simulink model "Parallel_n49"  (R2012b)
settings: Solver=VariableStepDiscrete  StartTime=0.0  StopTime=TotalIterations  RelTol=1e-3
values from neighbouring files (symbols this model uses):
  bp = 12    [ConfigValidate.m]
  bpSNMemory = bp    (= 12)    [ConfigValidate.m]
  IterationsOrdering = 4000    [ConfigValidate.m]
  MaxCoordDistance = (abs(max(wx) - min(wx))+abs(max(wy) - min(wy)))^2    [ConfigValidate.m]
  N_limit = 0.01    [ConfigValidate.m]
  nBits = 9    [ConfigValidate.m]
  nBitsNSmemories = (ceil(log2(TotalIterations)))    [ConfigValidate.m]
  S_limit = 1    [ConfigValidate.m]
  SourceNodes = 2000    [ConfigValidate.m]
  ts = 1    [ConfigValidate.m]
  w1 = rand(1,Neurons)    [ConfigValidate.m]
  w2 = rand(1,Neurons)    [ConfigValidate.m]
  wx = zeros(1,Neurons)    [ConfigValidate.m]
  wy = zeros(1,Neurons)    [ConfigValidate.m]
  x1 = rand(SourceNodes,1)    [ConfigValidate.m]
  x2 = rand(SourceNodes,1)    [ConfigValidate.m]
libraries: xbsIndex_r4 x4147, dspsrcs4 x2, dspstat3 x2
(part 2 of 19)

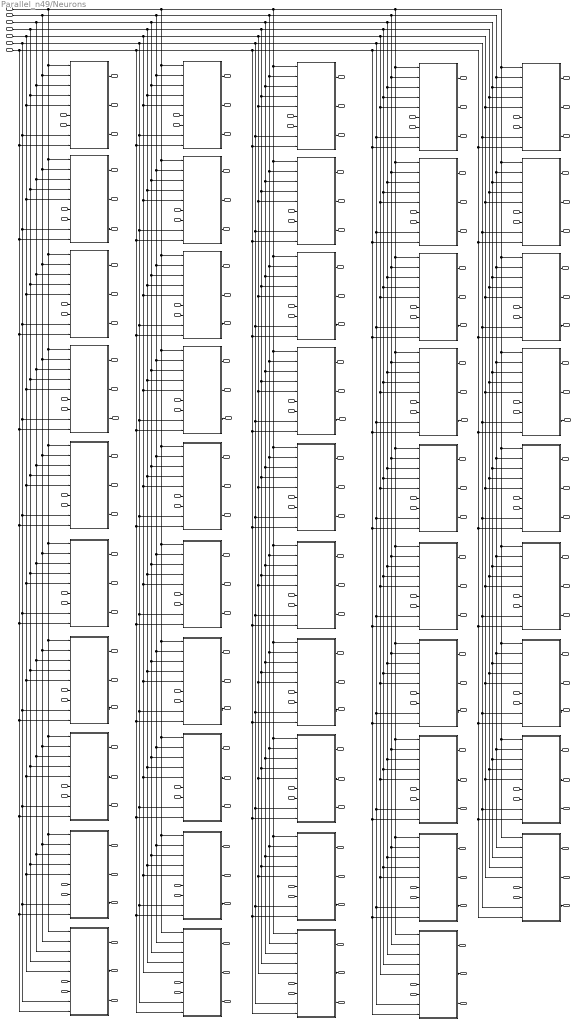
== system Parallel_n49/Neurons ==
  vX11 : Inport
  vX12 : Inport  Port=2
  S : Inport  Port=3
  N : Inport  Port=4
  memControl : Inport  Port=5
  wx_win : Inport  Port=6
  wy_win : Inport  Port=7
  wx1 : Inport  Port=8
  wy1 : Inport  Port=9
  wx2 : Inport  Port=10
  wy2 : Inport  Port=11
  wx3 : Inport  Port=12
  wy3 : Inport  Port=13
  wx4 : Inport  Port=14
  wy4 : Inport  Port=15
  wx5 : Inport  Port=16
  wy5 : Inport  Port=17
  wx6 : Inport  Port=18
  wy6 : Inport  Port=19
  wx7 : Inport  Port=20
  wy7 : Inport  Port=21
  wx8 : Inport  Port=22
  wy8 : Inport  Port=23
  wx9 : Inport  Port=24
  wy9 : Inport  Port=25
  wx10 : Inport  Port=26
  wy10 : Inport  Port=27
  wx11 : Inport  Port=28
  wy11 : Inport  Port=29
  wx12 : Inport  Port=30
  wy12 : Inport  Port=31
  wx13 : Inport  Port=32
  wy13 : Inport  Port=33
  wx14 : Inport  Port=34
  wy14 : Inport  Port=35
  wx15 : Inport  Port=36
  wy15 : Inport  Port=37
  wx16 : Inport  Port=38
  wy16 : Inport  Port=39
  wx17 : Inport  Port=40
  wy17 : Inport  Port=41
  wx18 : Inport  Port=42
  wy18 : Inport  Port=43
  wx19 : Inport  Port=44
  wy19 : Inport  Port=45
  wx20 : Inport  Port=46
  wy20 : Inport  Port=47
  wx21 : Inport  Port=48
  wy21 : Inport  Port=49
  wx22 : Inport  Port=50
  wy22 : Inport  Port=51
  wx23 : Inport  Port=52
  wy23 : Inport  Port=53
  wx24 : Inport  Port=54
  wy24 : Inport  Port=55
  wx25 : Inport  Port=56
  wy25 : Inport  Port=57
  wx26 : Inport  Port=58
  wy26 : Inport  Port=59
  wx27 : Inport  Port=60
  wy27 : Inport  Port=61
  wx28 : Inport  Port=62
  wy28 : Inport  Port=63
  wx29 : Inport  Port=64
  wy29 : Inport  Port=65
  wx30 : Inport  Port=66
  wy30 : Inport  Port=67
  wx31 : Inport  Port=68
  wy31 : Inport  Port=69
  wx32 : Inport  Port=70
  wy32 : Inport  Port=71
  wx33 : Inport  Port=72
  wy33 : Inport  Port=73
  wx34 : Inport  Port=74
  wy34 : Inport  Port=75
  wx35 : Inport  Port=76
  wy35 : Inport  Port=77
  wx36 : Inport  Port=78
  wy36 : Inport  Port=79
  wx37 : Inport  Port=80
  wy37 : Inport  Port=81
  wx38 : Inport  Port=82
  wy38 : Inport  Port=83
  wx39 : Inport  Port=84
  wy39 : Inport  Port=85
  wx40 : Inport  Port=86
  wy40 : Inport  Port=87
  wx41 : Inport  Port=88
  wy41 : Inport  Port=89
  wx42 : Inport  Port=90
  wy42 : Inport  Port=91
  wx43 : Inport  Port=92
  wy43 : Inport  Port=93
  wx44 : Inport  Port=94
  wy44 : Inport  Port=95
  wx45 : Inport  Port=96
  wy45 : Inport  Port=97
  wx46 : Inport  Port=98
  wy46 : Inport  Port=99
  wx47 : Inport  Port=100
  wy47 : Inport  Port=101
  wx48 : Inport  Port=102
  wy48 : Inport  Port=103
  wx49 : Inport  Port=104
  wy49 : Inport  Port=105
  Neuron1 : Subsystem
  Neuron10 : Subsystem
  Neuron11 : Subsystem
  Neuron12 : Subsystem
  Neuron13 : Subsystem
  Neuron14 : Subsystem
  Neuron15 : Subsystem
  Neuron16 : Subsystem
  Neuron17 : Subsystem
  Neuron18 : Subsystem
  Neuron19 : Subsystem
  Neuron2 : Subsystem
  Neuron20 : Subsystem
  Neuron21 : Subsystem
  Neuron22 : Subsystem
  Neuron23 : Subsystem
  Neuron24 : Subsystem
  Neuron25 : Subsystem
  Neuron26 : Subsystem
  Neuron27 : Subsystem
  Neuron28 : Subsystem
  Neuron29 : Subsystem
  Neuron3 : Subsystem
  Neuron30 : Subsystem
  Neuron31 : Subsystem
  Neuron32 : Subsystem
  Neuron33 : Subsystem
  Neuron34 : Subsystem
  Neuron35 : Subsystem
  Neuron36 : Subsystem
  Neuron37 : Subsystem
  Neuron38 : Subsystem
  Neuron39 : Subsystem
  Neuron4 : Subsystem
  Neuron40 : Subsystem
  Neuron41 : Subsystem
  Neuron42 : Subsystem
  Neuron43 : Subsystem
  Neuron44 : Subsystem
  Neuron45 : Subsystem
  Neuron46 : Subsystem
  Neuron47 : Subsystem
  Neuron48 : Subsystem
  Neuron49 : Subsystem
  Neuron5 : Subsystem
  Neuron6 : Subsystem
  Neuron7 : Subsystem
  Neuron8 : Subsystem
  Neuron9 : Subsystem
  w1n1 : Outport
  w1n2 : Outport  Port=2
  w1n3 : Outport  Port=3
  w1n4 : Outport  Port=4
  w1n5 : Outport  Port=5
  w1n6 : Outport  Port=6
  w1n7 : Outport  Port=7
  w1n8 : Outport  Port=8
  w1n9 : Outport  Port=9
  w1n10 : Outport  Port=10
  w1n11 : Outport  Port=11
  w1n12 : Outport  Port=12
  w1n13 : Outport  Port=13
  w1n14 : Outport  Port=14
  w1n15 : Outport  Port=15
  w1n16 : Outport  Port=16
  w1n17 : Outport  Port=17
  w1n18 : Outport  Port=18
  w1n19 : Outport  Port=19
  w1n20 : Outport  Port=20
  w1n21 : Outport  Port=21
  w1n22 : Outport  Port=22
  w1n23 : Outport  Port=23
  w1n24 : Outport  Port=24
  w1n25 : Outport  Port=25
  w1n26 : Outport  Port=26
  w1n27 : Outport  Port=27
  w1n28 : Outport  Port=28
  w1n29 : Outport  Port=29
  w1n30 : Outport  Port=30
  w1n31 : Outport  Port=31
  w1n32 : Outport  Port=32
  w1n33 : Outport  Port=33
  w1n34 : Outport  Port=34
  w1n35 : Outport  Port=35
  w1n36 : Outport  Port=36
  w1n37 : Outport  Port=37
  w1n38 : Outport  Port=38
  w1n39 : Outport  Port=39
  w1n40 : Outport  Port=40
  w1n41 : Outport  Port=41
  w1n42 : Outport  Port=42
  w1n43 : Outport  Port=43
  w1n44 : Outport  Port=44
  w1n45 : Outport  Port=45
  w1n46 : Outport  Port=46
  w1n47 : Outport  Port=47
  w1n48 : Outport  Port=48
  w1n49 : Outport  Port=49
  w2n1 : Outport  Port=50
  w2n2 : Outport  Port=51
  w2n3 : Outport  Port=52
  w2n4 : Outport  Port=53
  w2n5 : Outport  Port=54
  w2n6 : Outport  Port=55
  w2n7 : Outport  Port=56
  w2n8 : Outport  Port=57
  w2n9 : Outport  Port=58
  w2n10 : Outport  Port=59
  w2n11 : Outport  Port=60
  w2n12 : Outport  Port=61
  w2n13 : Outport  Port=62
  w2n14 : Outport  Port=63
  w2n15 : Outport  Port=64
  w2n16 : Outport  Port=65
  w2n17 : Outport  Port=66
  w2n18 : Outport  Port=67
  w2n19 : Outport  Port=68
  w2n20 : Outport  Port=69
  w2n21 : Outport  Port=70
  w2n22 : Outport  Port=71
  w2n23 : Outport  Port=72
  w2n24 : Outport  Port=73
  w2n25 : Outport  Port=74
  w2n26 : Outport  Port=75
  w2n27 : Outport  Port=76
  w2n28 : Outport  Port=77
  w2n29 : Outport  Port=78
  w2n30 : Outport  Port=79
  w2n31 : Outport  Port=80
  w2n32 : Outport  Port=81
  w2n33 : Outport  Port=82
  w2n34 : Outport  Port=83
  w2n35 : Outport  Port=84
  w2n36 : Outport  Port=85
  w2n37 : Outport  Port=86
  w2n38 : Outport  Port=87
  w2n39 : Outport  Port=88
  w2n40 : Outport  Port=89
  w2n41 : Outport  Port=90
  w2n42 : Outport  Port=91
  w2n43 : Outport  Port=92
  w2n44 : Outport  Port=93
  w2n45 : Outport  Port=94
  w2n46 : Outport  Port=95
  w2n47 : Outport  Port=96
  w2n48 : Outport  Port=97
  w2n49 : Outport  Port=98
  dist_n1 : Outport  Port=99
  dist_n2 : Outport  Port=100
  dist_n3 : Outport  Port=101
  dist_n4 : Outport  Port=102
  dist_n5 : Outport  Port=103
  dist_n6 : Outport  Port=104
  dist_n7 : Outport  Port=105
  dist_n8 : Outport  Port=106
  dist_n9 : Outport  Port=107
  dist_n10 : Outport  Port=108
  dist_n11 : Outport  Port=109
  dist_n12 : Outport  Port=110
  dist_n13 : Outport  Port=111
  dist_n14 : Outport  Port=112
  dist_n15 : Outport  Port=113
  dist_n16 : Outport  Port=114
  dist_n17 : Outport  Port=115
  dist_n18 : Outport  Port=116
  dist_n19 : Outport  Port=117
  dist_n20 : Outport  Port=118
  dist_n21 : Outport  Port=119
  dist_n22 : Outport  Port=120
  dist_n23 : Outport  Port=121
  dist_n24 : Outport  Port=122
  dist_n25 : Outport  Port=123
  dist_n26 : Outport  Port=124
  dist_n27 : Outport  Port=125
  dist_n28 : Outport  Port=126
  dist_n29 : Outport  Port=127
  dist_n30 : Outport  Port=128
  dist_n31 : Outport  Port=129
  dist_n32 : Outport  Port=130
  dist_n33 : Outport  Port=131
  dist_n34 : Outport  Port=132
  dist_n35 : Outport  Port=133
  dist_n36 : Outport  Port=134
  dist_n37 : Outport  Port=135
  dist_n38 : Outport  Port=136
  dist_n39 : Outport  Port=137
  dist_n40 : Outport  Port=138
  dist_n41 : Outport  Port=139
  dist_n42 : Outport  Port=140
  dist_n43 : Outport  Port=141
  dist_n44 : Outport  Port=142
  dist_n45 : Outport  Port=143
  dist_n46 : Outport  Port=144
  dist_n47 : Outport  Port=145
  dist_n48 : Outport  Port=146
  dist_n49 : Outport  Port=147
  wires:
  wy1/1 -> Neuron1/7(wy_n1)
  Neuron2/1(w1-n1) -> w1n2/1
  Neuron1/1(w1-n1) -> w1n1/1
  wy3/1 -> Neuron3/7(wy_n1)
  wy2/1 -> Neuron2/7(wy_n1)
  Neuron3/1(w1-n1) -> w1n3/1
  wx3/1 -> Neuron3/6(wx_n1)
  wx2/1 -> Neuron2/6(wx_n1)
  wy4/1 -> Neuron4/7(wy_n1)
  wx4/1 -> Neuron4/6(wx_n1)
  Neuron4/1(w1-n1) -> w1n4/1
  wy5/1 -> Neuron5/7(wy_n1)
  wx5/1 -> Neuron5/6(wx_n1)
  wy6/1 -> Neuron6/7(wy_n1)
  wx6/1 -> Neuron6/6(wx_n1)
  wy7/1 -> Neuron7/7(wy_n1)
  wx7/1 -> Neuron7/6(wx_n1)
  wy8/1 -> Neuron8/7(wy_n1)
  wx8/1 -> Neuron8/6(wx_n1)
  wy9/1 -> Neuron9/7(wy_n1)
  wx9/1 -> Neuron9/6(wx_n1)
  wy10/1 -> Neuron10/7(wy_n1)
  wx10/1 -> Neuron10/6(wx_n1)
  wy11/1 -> Neuron11/7(wy_n1)
  wx11/1 -> Neuron11/6(wx_n1)
  wy12/1 -> Neuron12/7(wy_n1)
  wx12/1 -> Neuron12/6(wx_n1)
  wy13/1 -> Neuron13/7(wy_n1)
  wx13/1 -> Neuron13/6(wx_n1)
  wy14/1 -> Neuron14/7(wy_n1)
  wx14/1 -> Neuron14/6(wx_n1)
  wy15/1 -> Neuron15/7(wy_n1)
  wx15/1 -> Neuron15/6(wx_n1)
  wy16/1 -> Neuron16/7(wy_n1)
  wx16/1 -> Neuron16/6(wx_n1)
  wy17/1 -> Neuron17/7(wy_n1)
  wx17/1 -> Neuron17/6(wx_n1)
  wy18/1 -> Neuron18/7(wy_n1)
  wx18/1 -> Neuron18/6(wx_n1)
  wy19/1 -> Neuron19/7(wy_n1)
  wx19/1 -> Neuron19/6(wx_n1)
  wy20/1 -> Neuron20/7(wy_n1)
  wx20/1 -> Neuron20/6(wx_n1)
  wy21/1 -> Neuron21/7(wy_n1)
  wx21/1 -> Neuron21/6(wx_n1)
  wy22/1 -> Neuron22/7(wy_n1)
  wx22/1 -> Neuron22/6(wx_n1)
  wy23/1 -> Neuron23/7(wy_n1)
  wx23/1 -> Neuron23/6(wx_n1)
  wy24/1 -> Neuron24/7(wy_n1)
  wx24/1 -> Neuron24/6(wx_n1)
  wy25/1 -> Neuron25/7(wy_n1)
  wx25/1 -> Neuron25/6(wx_n1)
  Neuron5/1(w1-n1) -> w1n5/1
  Neuron6/1(w1-n1) -> w1n6/1
  Neuron7/1(w1-n1) -> w1n7/1
  Neuron8/1(w1-n1) -> w1n8/1
  Neuron9/1(w1-n1) -> w1n9/1
  Neuron10/1(w1-n1) -> w1n10/1
  Neuron11/1(w1-n1) -> w1n11/1
  Neuron12/1(w1-n1) -> w1n12/1
  Neuron13/1(w1-n1) -> w1n13/1
  Neuron14/1(w1-n1) -> w1n14/1
  Neuron15/1(w1-n1) -> w1n15/1
  Neuron16/1(w1-n1) -> w1n16/1
  Neuron17/1(w1-n1) -> w1n17/1
  Neuron18/1(w1-n1) -> w1n18/1
  Neuron19/1(w1-n1) -> w1n19/1
  Neuron20/1(w1-n1) -> w1n20/1
  Neuron21/1(w1-n1) -> w1n21/1
  Neuron22/1(w1-n1) -> w1n22/1
  Neuron23/1(w1-n1) -> w1n23/1
  Neuron24/1(w1-n1) -> w1n24/1
  Neuron25/1(w1-n1) -> w1n25/1
  wx1/1 -> Neuron1/6(wx_n1)
  wy26/1 -> Neuron26/7(wy_n1)
  wx26/1 -> Neuron26/6(wx_n1)
  wy27/1 -> Neuron27/7(wy_n1)
  wx27/1 -> Neuron27/6(wx_n1)
  wy28/1 -> Neuron28/7(wy_n1)
  wx28/1 -> Neuron28/6(wx_n1)
  wy29/1 -> Neuron29/7(wy_n1)
  wx29/1 -> Neuron29/6(wx_n1)
  wy30/1 -> Neuron30/7(wy_n1)
  wx30/1 -> Neuron30/6(wx_n1)
  Neuron26/1(w1-n1) -> w1n26/1
  Neuron27/1(w1-n1) -> w1n27/1
  Neuron28/1(w1-n1) -> w1n28/1
  Neuron29/1(w1-n1) -> w1n29/1
  Neuron30/1(w1-n1) -> w1n30/1
  wy31/1 -> Neuron31/7(wy_n1)
  wx31/1 -> Neuron31/6(wx_n1)
  wy32/1 -> Neuron32/7(wy_n1)
  wx32/1 -> Neuron32/6(wx_n1)
  wy33/1 -> Neuron33/7(wy_n1)
  wx33/1 -> Neuron33/6(wx_n1)
  wy34/1 -> Neuron34/7(wy_n1)
  wx34/1 -> Neuron34/6(wx_n1)
  wy35/1 -> Neuron35/7(wy_n1)
  wx35/1 -> Neuron35/6(wx_n1)
  wy36/1 -> Neuron36/7(wy_n1)
  wx36/1 -> Neuron36/6(wx_n1)
  wy37/1 -> Neuron37/7(wy_n1)
  wx37/1 -> Neuron37/6(wx_n1)
  wy38/1 -> Neuron38/7(wy_n1)
  wx38/1 -> Neuron38/6(wx_n1)
  wy39/1 -> Neuron39/7(wy_n1)
  wx39/1 -> Neuron39/6(wx_n1)
  wy40/1 -> Neuron40/7(wy_n1)
  wx40/1 -> Neuron40/6(wx_n1)
  Neuron31/1(w1-n1) -> w1n31/1
  Neuron32/1(w1-n1) -> w1n32/1
  Neuron33/1(w1-n1) -> w1n33/1
  Neuron34/1(w1-n1) -> w1n34/1
  Neuron35/1(w1-n1) -> w1n35/1
  Neuron36/1(w1-n1) -> w1n36/1
  Neuron37/1(w1-n1) -> w1n37/1
  Neuron38/1(w1-n1) -> w1n38/1
  Neuron39/1(w1-n1) -> w1n39/1
  Neuron40/1(w1-n1) -> w1n40/1
  wy41/1 -> Neuron41/7(wy_n1)
  wx41/1 -> Neuron41/6(wx_n1)
  wy42/1 -> Neuron42/7(wy_n1)
  wx42/1 -> Neuron42/6(wx_n1)
  wy43/1 -> Neuron43/7(wy_n1)
  wx43/1 -> Neuron43/6(wx_n1)
  wy44/1 -> Neuron44/7(wy_n1)
  wx44/1 -> Neuron44/6(wx_n1)
  wy45/1 -> Neuron45/7(wy_n1)
  wx45/1 -> Neuron45/6(wx_n1)
  Neuron41/1(w1-n1) -> w1n41/1
  Neuron42/1(w1-n1) -> w1n42/1
  Neuron43/1(w1-n1) -> w1n43/1
  Neuron44/1(w1-n1) -> w1n44/1
  Neuron45/1(w1-n1) -> w1n45/1
  wy46/1 -> Neuron46/7(wy_n1)
  wx46/1 -> Neuron46/6(wx_n1)
  wy47/1 -> Neuron47/7(wy_n1)
  wx47/1 -> Neuron47/6(wx_n1)
  wy48/1 -> Neuron48/7(wy_n1)
  wx48/1 -> Neuron48/6(wx_n1)
  wy49/1 -> Neuron49/7(wy_n1)
  wx49/1 -> Neuron49/6(wx_n1)
  Neuron46/1(w1-n1) -> w1n46/1
  Neuron47/1(w1-n1) -> w1n47/1
  Neuron48/1(w1-n1) -> w1n48/1
  Neuron49/1(w1-n1) -> w1n49/1
  memControl/1 -> Neuron5/5(MemoryControl), Neuron45/5(MemoryControl), Neuron40/5(MemoryControl), Neuron35/5(MemoryControl), Neuron30/5(MemoryControl), Neuron25/5(MemoryControl), Neuron20/5(MemoryControl), Neuron15/5(MemoryControl), Neuron10/5(MemoryControl), Neuron9/5(MemoryControl), Neuron49/5(MemoryControl), Neuron44/5(MemoryControl), Neuron39/5(MemoryControl), Neuron34/5(MemoryControl), Neuron29/5(MemoryControl), Neuron24/5(MemoryControl), Neuron19/5(MemoryControl), Neuron14/5(MemoryControl), Neuron4/5(MemoryControl), Neuron48/5(MemoryControl), Neuron43/5(MemoryControl), Neuron38/5(MemoryControl), Neuron33/5(MemoryControl), Neuron28/5(MemoryControl), Neuron23/5(MemoryControl), Neuron18/5(MemoryControl), Neuron13/5(MemoryControl), Neuron8/5(MemoryControl), Neuron3/5(MemoryControl), Neuron47/5(MemoryControl), Neuron42/5(MemoryControl), Neuron37/5(MemoryControl), Neuron32/5(MemoryControl), Neuron27/5(MemoryControl), Neuron22/5(MemoryControl), Neuron17/5(MemoryControl), Neuron12/5(MemoryControl), Neuron7/5(MemoryControl), Neuron2/5(MemoryControl), Neuron46/5(MemoryControl), Neuron41/5(MemoryControl), Neuron36/5(MemoryControl), Neuron31/5(MemoryControl), Neuron26/5(MemoryControl), Neuron21/5(MemoryControl), Neuron16/5(MemoryControl), Neuron11/5(MemoryControl), Neuron6/5(MemoryControl), Neuron1/5(MemoryControl)
  S/1 -> Neuron45/3(S), Neuron40/3(S), Neuron35/3(S), Neuron30/3(S), Neuron25/3(S), Neuron20/3(S), Neuron15/3(S), Neuron10/3(S), Neuron5/3(S), Neuron49/3(S), Neuron44/3(S), Neuron39/3(S), Neuron34/3(S), Neuron29/3(S), Neuron24/3(S), Neuron19/3(S), Neuron14/3(S), Neuron9/3(S), Neuron4/3(S), Neuron13/3(S), Neuron48/3(S), Neuron43/3(S), Neuron38/3(S), Neuron33/3(S), Neuron28/3(S), Neuron23/3(S), Neuron18/3(S), Neuron8/3(S), Neuron3/3(S), Neuron7/3(S), Neuron47/3(S), Neuron42/3(S), Neuron37/3(S), Neuron32/3(S), Neuron27/3(S), Neuron22/3(S), Neuron17/3(S), Neuron12/3(S), Neuron2/3(S), Neuron46/3(S), Neuron41/3(S), Neuron36/3(S), Neuron31/3(S), Neuron26/3(S), Neuron21/3(S), Neuron16/3(S), Neuron11/3(S), Neuron6/3(S), Neuron1/3(S)
  N/1 -> Neuron45/4(N), Neuron40/4(N), Neuron35/4(N), Neuron30/4(N), Neuron25/4(N), Neuron20/4(N), Neuron15/4(N), Neuron10/4(N), Neuron5/4(N), Neuron49/4(N), Neuron44/4(N), Neuron39/4(N), Neuron34/4(N), Neuron29/4(N), Neuron24/4(N), Neuron19/4(N), Neuron14/4(N), Neuron9/4(N), Neuron4/4(N), Neuron48/4(N), Neuron43/4(N), Neuron38/4(N), Neuron33/4(N), Neuron28/4(N), Neuron23/4(N), Neuron18/4(N), Neuron13/4(N), Neuron8/4(N), Neuron3/4(N), Neuron47/4(N), Neuron42/4(N), Neuron37/4(N), Neuron32/4(N), Neuron27/4(N), Neuron22/4(N), Neuron17/4(N), Neuron12/4(N), Neuron7/4(N), Neuron2/4(N), Neuron46/4(N), Neuron41/4(N), Neuron36/4(N), Neuron31/4(N), Neuron26/4(N), Neuron21/4(N), Neuron16/4(N), Neuron11/4(N), Neuron6/4(N), Neuron1/4(N)
  vX12/1 -> Neuron45/2(vX12), Neuron40/2(vX12), Neuron35/2(vX12), Neuron30/2(vX12), Neuron25/2(vX12), Neuron20/2(vX12), Neuron15/2(vX12), Neuron10/2(vX12), Neuron5/2(vX12), Neuron49/2(vX12), Neuron44/2(vX12), Neuron39/2(vX12), Neuron34/2(vX12), Neuron29/2(vX12), Neuron24/2(vX12), Neuron19/2(vX12), Neuron14/2(vX12), Neuron9/2(vX12), Neuron4/2(vX12), Neuron48/2(vX12), Neuron43/2(vX12), Neuron38/2(vX12), Neuron33/2(vX12), Neuron28/2(vX12), Neuron23/2(vX12), Neuron18/2(vX12), Neuron13/2(vX12), Neuron8/2(vX12), Neuron3/2(vX12), Neuron12/2(vX12), Neuron47/2(vX12), Neuron42/2(vX12), Neuron37/2(vX12), Neuron32/2(vX12), Neuron27/2(vX12), Neuron22/2(vX12), Neuron17/2(vX12), Neuron7/2(vX12), Neuron2/2(vX12), Neuron46/2(vX12), Neuron41/2(vX12), Neuron36/2(vX12), Neuron31/2(vX12), Neuron26/2(vX12), Neuron21/2(vX12), Neuron16/2(vX12), Neuron11/2(vX12), Neuron6/2(vX12), Neuron1/2(vX12)
  vX11/1 -> Neuron4/1(vX11), Neuron49/1(vX11), Neuron44/1(vX11), Neuron39/1(vX11), Neuron34/1(vX11), Neuron29/1(vX11), Neuron24/1(vX11), Neuron19/1(vX11), Neuron14/1(vX11), Neuron9/1(vX11), Neuron45/1(vX11), Neuron40/1(vX11), Neuron35/1(vX11), Neuron30/1(vX11), Neuron25/1(vX11), Neuron20/1(vX11), Neuron15/1(vX11), Neuron10/1(vX11), Neuron5/1(vX11), Neuron48/1(vX11), Neuron43/1(vX11), Neuron38/1(vX11), Neuron33/1(vX11), Neuron28/1(vX11), Neuron23/1(vX11), Neuron18/1(vX11), Neuron13/1(vX11), Neuron8/1(vX11), Neuron3/1(vX11), Neuron47/1(vX11), Neuron42/1(vX11), Neuron37/1(vX11), Neuron32/1(vX11), Neuron27/1(vX11), Neuron22/1(vX11), Neuron17/1(vX11), Neuron12/1(vX11), Neuron7/1(vX11), Neuron2/1(vX11), Neuron1/1(vX11), Neuron46/1(vX11), Neuron41/1(vX11), Neuron36/1(vX11), Neuron31/1(vX11), Neuron26/1(vX11), Neuron21/1(vX11), Neuron16/1(vX11), Neuron11/1(vX11), Neuron6/1(vX11)
  wx_win/1 -> Neuron49/8(wxWinningNeuron), Neuron44/8(wxWinningNeuron), Neuron39/8(wxWinningNeuron), Neuron34/8(wxWinningNeuron), Neuron29/8(wxWinningNeuron), Neuron24/8(wxWinningNeuron), Neuron19/8(wxWinningNeuron), Neuron14/8(wxWinningNeuron), Neuron9/8(wxWinningNeuron), Neuron4/8(wxWinningNeuron), Neuron45/8(wxWinningNeuron), Neuron40/8(wxWinningNeuron), Neuron35/8(wxWinningNeuron), Neuron30/8(wxWinningNeuron), Neuron25/8(wxWinningNeuron), Neuron20/8(wxWinningNeuron), Neuron15/8(wxWinningNeuron), Neuron10/8(wxWinningNeuron), Neuron5/8(wxWinningNeuron), Neuron48/8(wxWinningNeuron), Neuron43/8(wxWinningNeuron), Neuron38/8(wxWinningNeuron), Neuron33/8(wxWinningNeuron), Neuron28/8(wxWinningNeuron), Neuron23/8(wxWinningNeuron), Neuron18/8(wxWinningNeuron), Neuron13/8(wxWinningNeuron), Neuron8/8(wxWinningNeuron), Neuron3/8(wxWinningNeuron), Neuron47/8(wxWinningNeuron), Neuron42/8(wxWinningNeuron), Neuron37/8(wxWinningNeuron), Neuron32/8(wxWinningNeuron), Neuron27/8(wxWinningNeuron), Neuron22/8(wxWinningNeuron), Neuron17/8(wxWinningNeuron), Neuron12/8(wxWinningNeuron), Neuron7/8(wxWinningNeuron), Neuron2/8(wxWinningNeuron), Neuron46/8(wxWinningNeuron), Neuron41/8(wxWinningNeuron), Neuron36/8(wxWinningNeuron), Neuron31/8(wxWinningNeuron), Neuron26/8(wxWinningNeuron), Neuron21/8(wxWinningNeuron), Neuron16/8(wxWinningNeuron), Neuron11/8(wxWinningNeuron), Neuron6/8(wxWinningNeuron), Neuron1/8(wxWinningNeuron)
  wy_win/1 -> Neuron46/9(wyWinningNeuron), Neuron41/9(wyWinningNeuron), Neuron36/9(wyWinningNeuron), Neuron31/9(wyWinningNeuron), Neuron26/9(wyWinningNeuron), Neuron21/9(wyWinningNeuron), Neuron16/9(wyWinningNeuron), Neuron11/9(wyWinningNeuron), Neuron6/9(wyWinningNeuron), Neuron1/9(wyWinningNeuron), Neuron47/9(wyWinningNeuron), Neuron42/9(wyWinningNeuron), Neuron37/9(wyWinningNeuron), Neuron32/9(wyWinningNeuron), Neuron27/9(wyWinningNeuron), Neuron22/9(wyWinningNeuron), Neuron17/9(wyWinningNeuron), Neuron12/9(wyWinningNeuron), Neuron7/9(wyWinningNeuron), Neuron2/9(wyWinningNeuron), Neuron48/9(wyWinningNeuron), Neuron43/9(wyWinningNeuron), Neuron38/9(wyWinningNeuron), Neuron33/9(wyWinningNeuron), Neuron28/9(wyWinningNeuron), Neuron23/9(wyWinningNeuron), Neuron18/9(wyWinningNeuron), Neuron13/9(wyWinningNeuron), Neuron8/9(wyWinningNeuron), Neuron3/9(wyWinningNeuron), Neuron49/9(wyWinningNeuron), Neuron44/9(wyWinningNeuron), Neuron39/9(wyWinningNeuron), Neuron34/9(wyWinningNeuron), Neuron29/9(wyWinningNeuron), Neuron24/9(wyWinningNeuron), Neuron19/9(wyWinningNeuron), Neuron14/9(wyWinningNeuron), Neuron9/9(wyWinningNeuron), Neuron4/9(wyWinningNeuron), Neuron45/9(wyWinningNeuron), Neuron40/9(wyWinningNeuron), Neuron35/9(wyWinningNeuron), Neuron30/9(wyWinningNeuron), Neuron25/9(wyWinningNeuron), Neuron20/9(wyWinningNeuron), Neuron15/9(wyWinningNeuron), Neuron10/9(wyWinningNeuron), Neuron5/9(wyWinningNeuron)
  Neuron1/2(w2-n1) -> w2n1/1
  Neuron2/2(w2-n1) -> w2n2/1
  Neuron3/2(w2-n1) -> w2n3/1
  Neuron4/2(w2-n1) -> w2n4/1
  Neuron5/2(w2-n1) -> w2n5/1
  Neuron6/2(w2-n1) -> w2n6/1
  Neuron7/2(w2-n1) -> w2n7/1
  Neuron8/2(w2-n1) -> w2n8/1
  Neuron9/2(w2-n1) -> w2n9/1
  Neuron10/2(w2-n1) -> w2n10/1
  Neuron11/2(w2-n1) -> w2n11/1
  Neuron12/2(w2-n1) -> w2n12/1
  Neuron13/2(w2-n1) -> w2n13/1
  Neuron14/2(w2-n1) -> w2n14/1
  Neuron15/2(w2-n1) -> w2n15/1
  Neuron16/2(w2-n1) -> w2n16/1
  Neuron17/2(w2-n1) -> w2n17/1
  Neuron18/2(w2-n1) -> w2n18/1
  Neuron19/2(w2-n1) -> w2n19/1
  Neuron20/2(w2-n1) -> w2n20/1
  Neuron21/2(w2-n1) -> w2n21/1
  Neuron22/2(w2-n1) -> w2n22/1
  Neuron23/2(w2-n1) -> w2n23/1
  Neuron24/2(w2-n1) -> w2n24/1
  Neuron25/2(w2-n1) -> w2n25/1
  Neuron26/2(w2-n1) -> w2n26/1
  Neuron27/2(w2-n1) -> w2n27/1
  Neuron28/2(w2-n1) -> w2n28/1
  Neuron29/2(w2-n1) -> w2n29/1
  Neuron30/2(w2-n1) -> w2n30/1
  Neuron31/2(w2-n1) -> w2n31/1
  Neuron32/2(w2-n1) -> w2n32/1
  Neuron33/2(w2-n1) -> w2n33/1
  Neuron34/2(w2-n1) -> w2n34/1
  Neuron35/2(w2-n1) -> w2n35/1
  Neuron36/2(w2-n1) -> w2n36/1
  Neuron37/2(w2-n1) -> w2n37/1
  Neuron38/2(w2-n1) -> w2n38/1
  Neuron39/2(w2-n1) -> w2n39/1
  Neuron40/2(w2-n1) -> w2n40/1
  Neuron41/2(w2-n1) -> w2n41/1
  Neuron42/2(w2-n1) -> w2n42/1
  Neuron43/2(w2-n1) -> w2n43/1
  Neuron44/2(w2-n1) -> w2n44/1
  Neuron45/2(w2-n1) -> w2n45/1
  Neuron46/2(w2-n1) -> w2n46/1
  Neuron47/2(w2-n1) -> w2n47/1
  Neuron48/2(w2-n1) -> w2n48/1
  Neuron49/2(w2-n1) -> w2n49/1
  Neuron1/3(dist_n1) -> dist_n1/1
  Neuron2/3(dist_n1) -> dist_n2/1
  Neuron3/3(dist_n1) -> dist_n3/1
  Neuron4/3(dist_n1) -> dist_n4/1
  Neuron5/3(dist_n1) -> dist_n5/1
  Neuron6/3(dist_n1) -> dist_n6/1
  Neuron7/3(dist_n1) -> dist_n7/1
  Neuron8/3(dist_n1) -> dist_n8/1
  Neuron9/3(dist_n1) -> dist_n9/1
  Neuron10/3(dist_n1) -> dist_n10/1
  Neuron11/3(dist_n1) -> dist_n11/1
  Neuron12/3(dist_n1) -> dist_n12/1
  Neuron13/3(dist_n1) -> dist_n13/1
  Neuron14/3(dist_n1) -> dist_n14/1
  Neuron15/3(dist_n1) -> dist_n15/1
  Neuron16/3(dist_n1) -> dist_n16/1
  Neuron17/3(dist_n1) -> dist_n17/1
  Neuron18/3(dist_n1) -> dist_n18/1
  Neuron19/3(dist_n1) -> dist_n19/1
  Neuron20/3(dist_n1) -> dist_n20/1
  Neuron21/3(dist_n1) -> dist_n21/1
  Neuron22/3(dist_n1) -> dist_n22/1
  Neuron23/3(dist_n1) -> dist_n23/1
  Neuron24/3(dist_n1) -> dist_n24/1
  Neuron25/3(dist_n1) -> dist_n25/1
  Neuron26/3(dist_n1) -> dist_n26/1
  Neuron27/3(dist_n1) -> dist_n27/1
  Neuron28/3(dist_n1) -> dist_n28/1
  Neuron29/3(dist_n1) -> dist_n29/1
  Neuron30/3(dist_n1) -> dist_n30/1
  Neuron31/3(dist_n1) -> dist_n31/1
  Neuron32/3(dist_n1) -> dist_n32/1
  Neuron33/3(dist_n1) -> dist_n33/1
  Neuron34/3(dist_n1) -> dist_n34/1
  Neuron35/3(dist_n1) -> dist_n35/1
  Neuron36/3(dist_n1) -> dist_n36/1
  Neuron37/3(dist_n1) -> dist_n37/1
  Neuron38/3(dist_n1) -> dist_n38/1
  Neuron39/3(dist_n1) -> dist_n39/1
  Neuron40/3(dist_n1) -> dist_n40/1
  Neuron41/3(dist_n1) -> dist_n41/1
  Neuron42/3(dist_n1) -> dist_n42/1
  Neuron43/3(dist_n1) -> dist_n43/1
  Neuron44/3(dist_n1) -> dist_n44/1
  Neuron45/3(dist_n1) -> dist_n45/1
  Neuron46/3(dist_n1) -> dist_n46/1
  Neuron47/3(dist_n1) -> dist_n47/1
  Neuron48/3(dist_n1) -> dist_n48/1
  Neuron49/3(dist_n1) -> dist_n49/1

== system Parallel_n49/TimeSeries_Functions ==
  note: Neighbor Function.
      | In the memory is stored the result of 1/2S² considering that S start from sqrt(neurons) and decrease to 1 (minimum value).
      | To avoid execute a divisor circuit inside the FPGA, in the memory is already stored the result of the division 1/2S² instead of stores only S
  note: Learning Function
      | The learning rate descreases from 0.1 to 0.001 during
      | ordering phase. In the covergence phase stays at the minimum.
  note: This circuits prevents all the memories in the circuit from working in the first clock cycle.
      | This helps prevent a response for a input equal to 1 in the beggining of the process.
  note: Note that the selector circuits in the memories are used to prevent the values
      | being less than the minimum value of each parameter during the ordering phase.
      | During the covergence phase it forces the minimum value
  Display{1..6} (6 alike) : Display
  DistMenor1 : xbsIndex_r4/Mux  inputs=2  en=off  latency=dMUX_CooperatingProcess  precision=Full  arith_type=Unsigned  n_bits=16  bin_pt=14  quantization=Truncate  overflow=Wrap  dbl_ovrd=off  block_type=mux
  DistMenor2 : xbsIndex_r4/Mux  inputs=2  en=off  latency=dMUX_CooperatingProcess  precision=Full  arith_type=Unsigned  n_bits=16  bin_pt=14  quantization=Truncate  overflow=Wrap  dbl_ovrd=off  block_type=mux
  Dist_compare1 : xbsIndex_r4/Relational  mode=a<=b  en=off  latency=dComparator_CooperatingProcess  dbl_ovrd=off  block_type=relational
  Dist_compare2 : xbsIndex_r4/Relational  mode=a>b  en=off  latency=dComparator_CooperatingProcess  dbl_ovrd=off  block_type=relational
  Dist_compare3 : xbsIndex_r4/Relational  mode=a>b  en=off  latency=dComparator_CooperatingProcess  dbl_ovrd=off  block_type=relational
  Dist_compare4 : xbsIndex_r4/Relational  mode=a=b  en=off  latency=dComparator_CooperatingProcess  dbl_ovrd=off  block_type=relational
  Gateway Out{1..6} (6 alike) : xbsIndex_r4/Gateway Out  inherit_from_input=off  hdl_port=off  timing_constraint=None  locs_specified=off  LOCs={}  UseAsDAC=off  DACChannel='1'  block_type=gatewayout
  Inverter : xbsIndex_r4/Inverter  en=off  latency=dInverter_CooperatingProcess  dbl_ovrd=off  block_type=inv
  LearningRateLimit : xbsIndex_r4/Constant  const=N_limit  gui_display_data_type=Fixed-point  arith_type=Signed (2's comp)  n_bits=bpSNMemory+1  bin_pt=bpSNMemory  preci_type=Single  exp_width=8  frac_width=24  explicit_period=on  period=ts  equ=P=C  opselect=C  inp2=PCIN>>17  opr=+  inp1=P  carry=CIN  dbl_ovrd=off  block_type=constant
  Learning_Rate : xbsIndex_r4/ROM  depth=2^nBitsNSmemories  initVector=N  distributed_mem=Block RAM  rst=off  init_reg=0  en=off  latency=dMemoryLearning  gui_display_data_type=Fixed-point  arith_type="Signed  (2's comp)"  n_bits=bpSNMemory+1  bin_pt=bpSNMemory  preci_type=Single  exp_width=8  frac_width=24  dbl_ovrd=off  optimize=Area  use_rpm=on  block_type=sprom
  Logical1 : xbsIndex_r4/Logical  logical_function=OR  inputs=2  en=off  latency=dOR_CooperatingProcess  precision=Full  arith_type=Unsigned  n_bits=16  bin_pt=0  align_bp=on  dbl_ovrd=off  block_type=logical
  Logical2 : xbsIndex_r4/Logical  logical_function=OR  inputs=2  en=off  latency=dOR_CooperatingProcess  precision=Full  arith_type=Unsigned  n_bits=16  bin_pt=0  align_bp=on  dbl_ovrd=off  block_type=logical
  Logical3 : xbsIndex_r4/Logical  logical_function=OR  inputs=2  en=off  latency=dAnd_CooperatingProcess  precision=Full  arith_type=Unsigned  n_bits=16  bin_pt=0  align_bp=on  dbl_ovrd=off  block_type=logical
  Neighborhood_Size : xbsIndex_r4/ROM  depth=2^nBitsNSmemories  initVector=S  distributed_mem=Block RAM  rst=off  init_reg=0  en=off  latency=dMemoryNeighbor  gui_display_data_type=Fixed-point  arith_type="Signed  (2's comp)"  n_bits=bpSNMemory+1  bin_pt=bpSNMemory  preci_type=Single  exp_width=8  frac_width=24  dbl_ovrd=off  optimize=Area  use_rpm=on  block_type=sprom
  Neighborhood_Size_Limit : xbsIndex_r4/Constant  const=S_limit  gui_display_data_type=Fixed-point  arith_type=Signed (2's comp)  n_bits=bpSNMemory+1  bin_pt=bpSNMemory  preci_type=Single  exp_width=8  frac_width=24  explicit_period=on  period=ts  equ=P=C  opselect=C  inp2=PCIN>>17  opr=+  inp1=P  carry=CIN  dbl_ovrd=off  block_type=constant
  OrderingPhase_offset : xbsIndex_r4/Constant  const=IterationsOrdering  gui_display_data_type=Fixed-point  arith_type=Unsigned  n_bits=12  bin_pt=0  preci_type=Single  exp_width=8  frac_width=24  explicit_period=on  period=ts  equ=P=C  opselect=C  inp2=PCIN>>17  opr=+  inp1=P  carry=CIN  dbl_ovrd=off  block_type=constant
  To Workspace : ToWorkspace  VariableName=S_histH  SampleTime=ts
  To Workspace1 : ToWorkspace  VariableName=N_histH  SampleTime=ts
  ZeroConstant : xbsIndex_r4/Constant  const=0  gui_display_data_type=Fixed-point  arith_type=Signed (2's comp)  n_bits=bpSNMemory+1  bin_pt=bpSNMemory  preci_type=Single  exp_width=8  frac_width=24  explicit_period=on  period=ts  equ=P=C  opselect=C  inp2=PCIN>>17  opr=+  inp1=P  carry=CIN  dbl_ovrd=off  block_type=constant
  count_reset : xbsIndex_r4/Counter  cnt_type=Free Running  cnt_to=(2^nBitsNSmemories)-1  operation=Up  start_count=0  cnt_by_val=1  arith_type=Unsigned  n_bits=nBitsNSmemories  bin_pt=0  load_pin=off  rst=off  en=on  explicit_period=on  period=ts  dbl_ovrd=off  use_behavioral_HDL=off  implementation=Fabric  block_type=counter
  delay_vX1 : xbsIndex_r4/Register  init=N_limit  rst=off  en=off  dbl_ovrd=off  block_type=register
  enable_bit : xbsIndex_r4/Constant  const=1  gui_display_data_type=Boolean  arith_type=Boolean  n_bits=nb  bin_pt=bp  preci_type=Single  exp_width=8  frac_width=24  explicit_period=on  period=ts  equ=P=C  opselect=C  inp2=PCIN>>17  opr=+  inp1=P  carry=CIN  dbl_ovrd=off  block_type=constant
  w1n1 : xbsIndex_r4/Register  init=0  rst=off  en=on  dbl_ovrd=off  block_type=register
  S : Outport
  N : Outport  Port=2
  MemControl : Outport  Port=3
  wires:
  w1n1/1 -> count_reset/1, MemControl/1, Inverter/1
  Inverter/1 -> w1n1/2
  enable_bit/1 -> w1n1/1
  DistMenor1/1 -> delay_vX1/1, Gateway Out6/1
  Gateway Out6/1 -> Display4/1, To Workspace1/1
  count_reset/1 -> Learning_Rate/1, Gateway Out4/1, Dist_compare3/1, Neighborhood_Size/1
  LearningRateLimit/1 -> DistMenor1/3, Dist_compare1/2
  Gateway Out5/1 -> To Workspace/1, Display3/1
  Neighborhood_Size/1 -> DistMenor2/2, Dist_compare2/1, Dist_compare4/1
  DistMenor2/1 -> S/1, Gateway Out5/1
  OrderingPhase_offset/1 -> Dist_compare3/2
  Dist_compare3/1 -> Logical1/1, Gateway Out1/1, Logical2/2
  Neighborhood_Size_Limit/1 -> DistMenor2/3, Dist_compare2/2
  Logical2/1 -> Gateway Out2/1, DistMenor2/1
  Logical1/1 -> Gateway Out3/1, DistMenor1/1
  Learning_Rate/1 -> DistMenor1/2, Dist_compare1/1
  Dist_compare1/1 -> Logical1/2
  Gateway Out1/1 -> Display1/1
  Gateway Out2/1 -> Display2/1
  Gateway Out3/1 -> Display5/1
  Gateway Out4/1 -> Display6/1
  Logical3/1 -> Logical2/1
  Dist_compare2/1 -> Logical3/2
  Dist_compare4/1 -> Logical3/1
  ZeroConstant/1 -> Dist_compare4/2
  delay_vX1/1 -> N/1
